simulink model "Rigid_Body_Simulation"  (R2016a)
settings: Solver=VariableStepAuto  StartTime=0.0  StopTime=10.0  RelTol=1e-3
libraries: lib_exmp x1
settings Model: Creator=devantormey  LastModifiedBy=devantormey

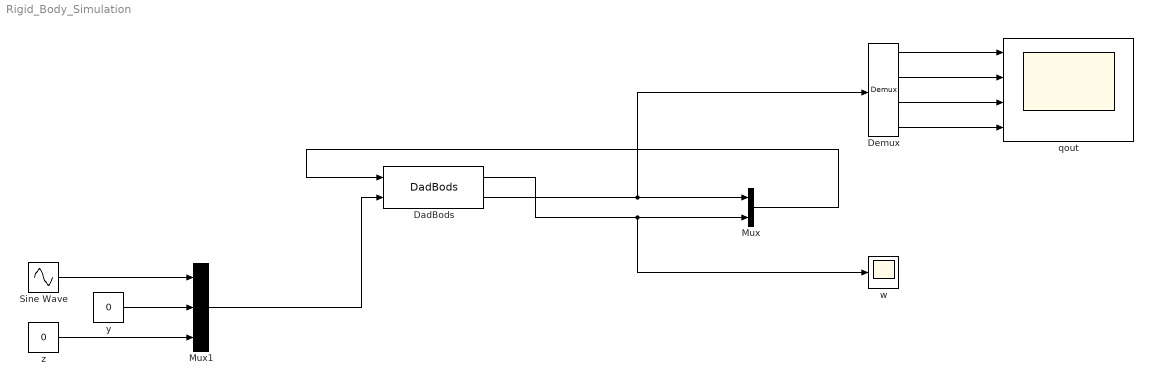
== system Rigid_Body_Simulation ==
  "DadBods " : lib_exmp/DadBods 
  Demux : Demux
  Mux : Mux  Inputs=2
  Mux1 : Mux  Inputs=3
  Sine Wave : Sin  Amplitude=.1  SampleTime=0
  qout : Scope  NumInputPorts=4
  w : Scope
  "y " : Constant  Value=0
  "z " : Constant  Value=0
  wires:
  "DadBods "/2 -> Demux/1, Mux/1
  "DadBods "/1 -> w/1, Mux/2
  Mux/1 -> "DadBods "/1
  Sine Wave/1 -> Mux1/1
  "y "/1 -> Mux1/2
  "z "/1 -> Mux1/3
  Mux1/1 -> "DadBods "/2
  Demux/1 -> qout/1
  Demux/2 -> qout/2
  Demux/3 -> qout/3
  Demux/4 -> qout/4
